simulink model "hinf_arduino_basic"  (R2015a)
settings: Solver=ode3  StartTime=0.0  StopTime=10.0  FixedStep=1/200  RelTol=1e-3
values from neighbouring files (symbols this model uses):
  Hinf = ss(Hinf_red)    [controller_parameters.m]
libraries: PoliArd x10
settings Model: ExtModeTrigDuration=2  Creator=User  LastModifiedBy=user
settings OptimizationCC: OptimizeModelRefInitCode=on  LifeSpan=1
settings DebuggingCC: UnderspecifiedInitializationDetection=Classic  MergeDetectMultiDrivingBlocksExec=none
settings HardwareCC: ProdLargestAtomicInteger=Long  ProdLargestAtomicFloat=Double  ProdEndianess=LittleEndian  ProdHWDeviceType=ARM Compatible->ARM Cortex
settings RTWCC: SystemTargetFile=realtime.tlc  GenerateMakefile=off  TemplateMakefile=realtime.tmf  Description=Run on Target Hardware  RTWVerbose=off
settings ERTTargetCC: CombineOutputUpdateFcns=off  ExtModeTransport=3  ExtModeMexFile=ext_serial_win32_comm_rtt  ExtModeMexArgs=0 1 9600  ERTSrcFileBannerTemplate=realtime_code_template.cgt  ERTHdrFileBannerTemplate=realtime_code_template.cgt  ERTDataSrcFileTemplate=realtime_code_template.cgt  ERTDataHdrFileTemplate=realtime_code_template.cgt  ERTCustomFileTemplate=realtime_file_process.tlc

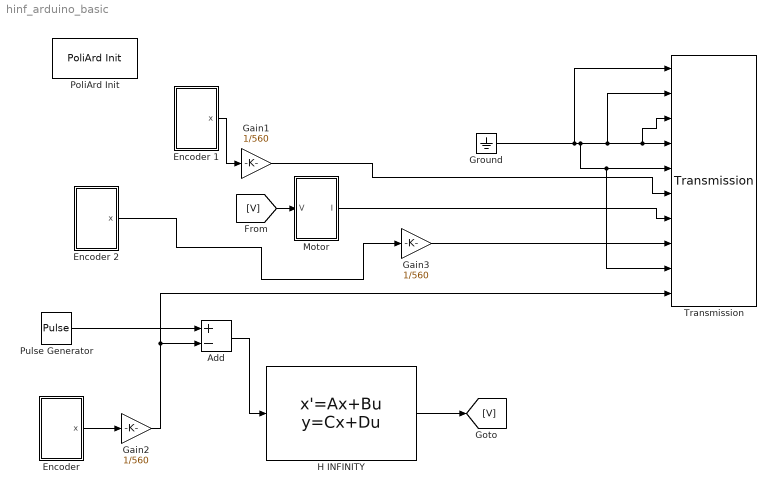
== system hinf_arduino_basic ==
  Add : Sum  Inputs=+-
  "Encoder " : Subsystem
  Encoder 1 : Subsystem
  Encoder 2 : Subsystem
  Gain1 : Gain  Gain=1/560
  Gain2 : Gain  Gain=1/560
  Gain3 : Gain  Gain=1/560
  Ground : Ground
  H INFINITY : StateSpace  A=Hinf.A  B=Hinf.B  C=Hinf.C  D=Hinf.D  X0=0
  Motor : Subsystem
  PoliArd Init : PoliArd/PoliArd Init
  Pulse Generator : DiscretePulseGenerator  PulseType=Time based  Amplitude=2  Period=10  PulseWidth=50  PhaseDelay=3
  Transmission : PoliArd/Transmission  sample_freq=200  sig_to_send=6
  wires:
  Ground/1 -> Transmission/1, Transmission/9, Transmission/5, Transmission/2, Transmission/3, Transmission/4
  Motor/1(I) -> Transmission/7
  "Encoder "/1(x) -> Gain2/1
  Gain2/1 -> Transmission/10, Add/2
  Encoder 1/1(x) -> Gain1/1
  Gain1/1 -> Transmission/6
  Gain3/1 -> Transmission/8
  Encoder 2/1(x) -> Gain3/1
  H INFINITY/1 -> [V]
  [V] -> Motor/1(V)
  Add/1 -> H INFINITY/1
  Pulse Generator/1 -> Add/1

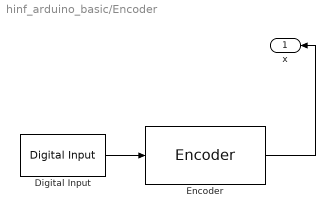
== system hinf_arduino_basic/Encoder  ==
  Digital Input : PoliArd/Digital Input  DI_pin=2  DIsample=1/200
  Encoder : PoliArd/Encoder  EncoderID=4  dt_enc=-1
  x : Outport
  wires:
  Digital Input/1 -> Encoder/1
  Encoder/1 -> x/1

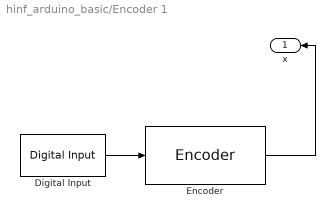
== system hinf_arduino_basic/Encoder 1 ==
  Digital Input : PoliArd/Digital Input  DI_pin=2  DIsample=1/200
  Encoder : PoliArd/Encoder  EncoderID=3  dt_enc=-1
  x : Outport
  wires:
  Digital Input/1 -> Encoder/1
  Encoder/1 -> x/1

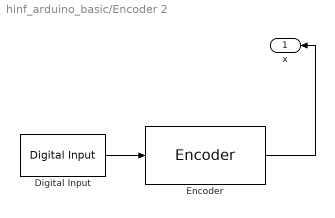
== system hinf_arduino_basic/Encoder 2 ==
  Digital Input : PoliArd/Digital Input  DI_pin=2  DIsample=1/200
  Encoder : PoliArd/Encoder  EncoderID=1  dt_enc=-1
  x : Outport
  wires:
  Digital Input/1 -> Encoder/1
  Encoder/1 -> x/1

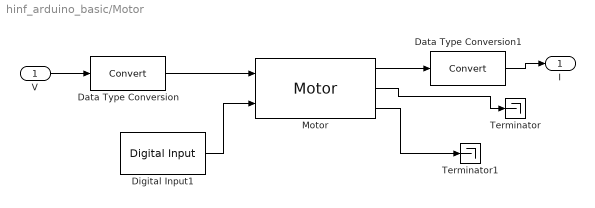
== system hinf_arduino_basic/Motor ==
  V : Inport
  Data Type Conversion : DataTypeConversion
  Data Type Conversion1 : DataTypeConversion
  Digital Input1 : PoliArd/Digital Input  DI_pin=3  DIsample=1/200
  Motor : PoliArd/Motor  MotorID=2  DC_bus_mask=12  dt_mot=1/200
  Terminator : Terminator
  Terminator1 : Terminator
  I : Outport
  wires:
  Data Type Conversion/1 -> Motor/1
  Digital Input1/1 -> Motor/2
  V/1 -> Data Type Conversion/1
  Motor/3 -> Terminator1/1
  Motor/2 -> Terminator/1
  Motor/1 -> Data Type Conversion1/1
  Data Type Conversion1/1 -> I/1
